simulink model "SimulinkLR3"  (R2016a)
settings: Solver=VariableStepAuto  StartTime=0.0  StopTime=0.1  RelTol=1e-3
values from neighbouring files (symbols this model uses):
  A = 0.5E-3    (= 0.0005)    [LR3.m]
  df = 1    [LR3.m]
  dFo = 5    [LR3.m]
  dt = 1E-4    (= 0.0001)    [LR3.m]
  f = Fo+Fd    (= 1991.8)    [LR3.m]
  f_op = zeros(N,1)    [LR3.m]
  Fo = 1990.0    (= 1990)    [LR3.m]
  sigma = sigmamass(5)    [LR3.m]
undefined symbols (not defined in the file or in its folder): DiscIntNeverNeededParam
libraries: dspstat3 x1, dspsrcs4 x1
settings Model: Creator=Энверыч  LastModifiedBy=Энверыч

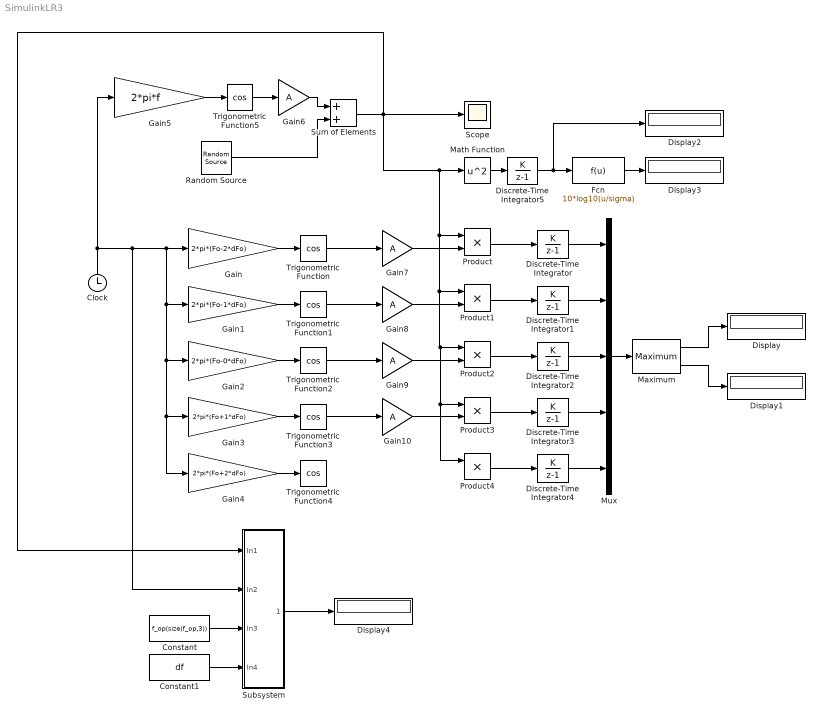
== system SimulinkLR3 ==
  Clock : Clock
  Constant : Constant  Value=f_op(size(f_op,3))
  Constant1 : Constant  Value=df
  Discrete-Time Integrator{,1..5} (6 alike) : DiscreteIntegrator  IntegratorMethod=Accumulation: Forward Euler  InitialConditionSetting=State (most efficient)  SampleTime=dt  ICPrevOutput=DiscIntNeverNeededParam  ICPrevScaledInput=DiscIntNeverNeededParam
  Display{,1..4} (5 alike) : Display
  Fcn : Fcn  Expr=10*log10(u/sigma)
  Gain : Gain  Gain=2*pi*(Fo-2*dFo)
  Gain1 : Gain  Gain=2*pi*(Fo-1*dFo)
  Gain{6..10} (5 alike) : Gain  Gain=A
  Gain2 : Gain  Gain=2*pi*(Fo-0*dFo)
  Gain3 : Gain  Gain=2*pi*(Fo+1*dFo)
  Gain4 : Gain  Gain=2*pi*(Fo+2*dFo)
  Gain5 : Gain  Gain=2*pi*f
  Math Function : Math  Operator=square  SaturateOnIntegerOverflow=on
  Maximum : dspstat3/Maximum  fcn=Value and Index  reset=None  InputProcessing=Columns as channels (frame based)  indexBase=One  operateOver=Each column  Dimension=1  operation=maximum  roiEnable=off  roiType=Rectangles  roiPortion=Entire ROI  roiOutput=Individual statistics for each ROI  roiFlag=off  accumDataTypeStr=Inherit: Same as product output  accumLastDataTypeStr=Inherit: Same as product output  roundingMode=Floor  overflowMode=off
  Mux : Mux  Inputs=5
  Product{,1..4} (5 alike) : Product
  Random Source : dspsrcs4/Random Source  SrcType=Gaussian  NormMethod=Ziggurat  CltLength=12  MinVal=0  MaxVal=1  MeanVal=0  VarVal=sigma^2  RepMode=Not repeatable  rawSeed=1  IsInherit=off  SampMode=Discrete  SampTime=dt  SampFrame=1  DataType=Double  OutComplex=Real  OutputFrames=off
  Scope : Scope
  Subsystem : Subsystem
  Sum of Elements : Sum
  Trigonometric Function{,1..5} (6 alike) : Trigonometry  Operator=cos
  wires:
  Gain/1 -> Trigonometric Function/1
  Gain1/1 -> Trigonometric Function1/1
  Gain2/1 -> Trigonometric Function2/1
  Gain3/1 -> Trigonometric Function3/1
  Gain4/1 -> Trigonometric Function4/1
  Clock/1 -> Gain5/1, Gain3/1, Gain4/1, Gain2/1, Gain1/1, Gain/1, Subsystem/2(In2)
  Gain5/1 -> Trigonometric Function5/1
  Random Source/1 -> Sum of Elements/2
  Product/1 -> Discrete-Time Integrator/1
  Product1/1 -> Discrete-Time Integrator1/1
  Product2/1 -> Discrete-Time Integrator2/1
  Product3/1 -> Discrete-Time Integrator3/1
  Product4/1 -> Discrete-Time Integrator4/1
  Discrete-Time Integrator/1 -> Mux/1
  Discrete-Time Integrator1/1 -> Mux/2
  Discrete-Time Integrator2/1 -> Mux/3
  Discrete-Time Integrator3/1 -> Mux/4
  Discrete-Time Integrator4/1 -> Mux/5
  Maximum/1 -> Display/1
  Maximum/2 -> Display1/1
  Mux/1 -> Maximum/1
  Math Function/1 -> Discrete-Time Integrator5/1
  Fcn/1 -> Display3/1
  Subsystem/1(Out1) -> Display4/1
  Sum of Elements/1 -> Subsystem/1(In1), Scope/1, Math Function/1, Product3/1, Product4/1, Product2/1, Product1/1, Product/1
  Constant1/1 -> Subsystem/4(In4)
  Constant/1 -> Subsystem/3(In3)
  Discrete-Time Integrator5/1 -> Display2/1, Fcn/1
  Trigonometric Function5/1 -> Gain6/1
  Gain6/1 -> Sum of Elements/1
  Trigonometric Function/1 -> Gain7/1
  Gain7/1 -> Product/2
  Trigonometric Function1/1 -> Gain8/1
  Gain8/1 -> Product1/2
  Trigonometric Function2/1 -> Gain9/1
  Trigonometric Function3/1 -> Gain10/1
  Gain9/1 -> Product2/2
  Gain10/1 -> Product3/2

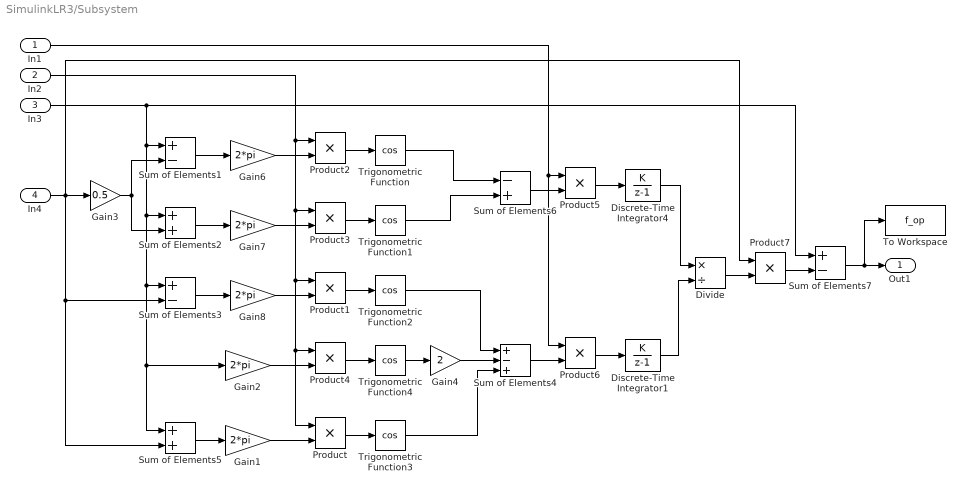
== system SimulinkLR3/Subsystem ==
  In1 : Inport
  In2 : Inport  Port=2
  In3 : Inport  Port=3
  In4 : Inport  Port=4
  Discrete-Time Integrator1 : DiscreteIntegrator  IntegratorMethod=Accumulation: Forward Euler  InitialConditionSetting=State (most efficient)  SampleTime=dt  ICPrevOutput=DiscIntNeverNeededParam  ICPrevScaledInput=DiscIntNeverNeededParam
  Discrete-Time Integrator4 : DiscreteIntegrator  IntegratorMethod=Accumulation: Forward Euler  InitialConditionSetting=State (most efficient)  SampleTime=dt  ICPrevOutput=DiscIntNeverNeededParam  ICPrevScaledInput=DiscIntNeverNeededParam
  Divide : Product  Inputs=*/
  Gain{1..2,6..8} (5 alike) : Gain  Gain=2*pi
  Gain3 : Gain  Gain=0.5
  Gain4 : Gain  Gain=2
  Product{,1..7} (8 alike) : Product
  Sum of Elements1 : Sum  Inputs=+-
  Sum of Elements2 : Sum
  Sum of Elements3 : Sum  Inputs=+-
  Sum of Elements4 : Sum  Inputs=+-+
  Sum of Elements5 : Sum
  Sum of Elements6 : Sum  Inputs=-+
  Sum of Elements7 : Sum  Inputs=+-
  To Workspace : ToWorkspace  VariableName=f_op  SampleTime=dt
  Trigonometric Function{,1..4} (5 alike) : Trigonometry  Operator=cos
  Out1 : Outport
  wires:
  Sum of Elements1/1 -> Gain6/1
  Sum of Elements2/1 -> Gain7/1
  Sum of Elements3/1 -> Gain8/1
  Sum of Elements5/1 -> Gain1/1
  Gain1/1 -> Product/2
  Gain8/1 -> Product1/2
  Gain6/1 -> Product2/2
  Gain7/1 -> Product3/2
  In2/1 -> Product2/1, Product3/1, Product/1, Product4/1, Product1/1
  Product2/1 -> Trigonometric Function/1
  Product/1 -> Trigonometric Function3/1
  Product1/1 -> Trigonometric Function2/1
  Product3/1 -> Trigonometric Function1/1
  Product4/1 -> Trigonometric Function4/1
  Gain2/1 -> Product4/2
  In3/1 -> Sum of Elements7/1, Gain2/1, Sum of Elements5/1, Sum of Elements3/1, Sum of Elements2/1, Sum of Elements1/1
  Gain3/1 -> Sum of Elements1/2, Sum of Elements2/2
  In4/1 -> Product7/1, Sum of Elements3/2, Sum of Elements5/2, Gain3/1
  Trigonometric Function4/1 -> Gain4/1
  Gain4/1 -> Sum of Elements4/2
  Trigonometric Function2/1 -> Sum of Elements4/1
  Trigonometric Function3/1 -> Sum of Elements4/3
  Trigonometric Function/1 -> Sum of Elements6/1
  Trigonometric Function1/1 -> Sum of Elements6/2
  Sum of Elements6/1 -> Product5/2
  In1/1 -> Product5/1, Product6/1
  Sum of Elements4/1 -> Product6/2
  Product5/1 -> Discrete-Time Integrator4/1
  Product6/1 -> Discrete-Time Integrator1/1
  Discrete-Time Integrator4/1 -> Divide/1
  Discrete-Time Integrator1/1 -> Divide/2
  Divide/1 -> Product7/2
  Product7/1 -> Sum of Elements7/2
  Sum of Elements7/1 -> To Workspace/1, Out1/1
